simulink model "sumiao_zed"  (R2019a)
settings: Solver=FixedStepDiscrete  StartTime=0.0  StopTime=402*320  RelTol=1e-3
undefined symbols (not defined in the file): HDTV, Rec, SDTV
libraries: simulink x7, visionzynq_privlib x3, visionhdlutilities x3, dspvision x1, visionhdlconversions x1, visionsinks x1, visionzynqlib x1
settings Model: DataTypeOverride=Off  SimulationMode=accelerator  Creator=lbai  LastModifiedBy=lbai
settings DataIOCC: LimitDataPoints=on  SaveOutput=off  SignalLogging=off  DSMLogging=off  VisualizeSimOutput=off  SaveTime=off
settings OptimizationCC: BlockReduction=off  ConditionallyExecuteInputs=off  DefaultParameterBehavior=Inlined  LifeSpan=inf  SimCompilerOptimization=on
settings DebuggingCC: AlgebraicLoopMsg=error  SingleTaskRateTransMsg=error  ParameterPrecisionLossMsg=none  AllowSymbolicDim=off  PregeneratedLibrarySubsystemCodeDiagnostic=none  SFUnexpectedBacktrackingDiag=warning  SFNoUnconditionalDefaultTransitionDiag=warning  SFExecutionAtInitializationDiag=none  IntegerSaturationMsg=none  ArithmeticOperatorsInVariantConditions=warning
settings HardwareCC: ProdBitPerPointer=32  ProdBitPerSizeT=32  ProdBitPerPtrDiffT=32  ProdLargestAtomicFloat=None  ProdIntDivRoundTo=Undefined  ProdEndianess=Unspecified  ProdWordSize=32  ProdHWDeviceType=ASIC/FPGA->ASIC/FPGA  ProdEqTarget=off
settings SFSimCC: SimUseLocalCustomCode=off
settings RTWCC: RTWUseLocalCustomCode=off  BuildConfiguration=Faster Runs
settings CodeAppCC: StateflowObjectComments=on
settings GRTTargetCC: TargetLangStandard=C89/C90 (ANSI)  GeneratePreprocessorConditionals=Disable all
settings ConfigComp: CovMetricSettings=dw  CovHtmlReporting=on  CovSaveCumulativeToWorkspaceVar=on  CovSaveSingleToWorkspaceVar=on  CovExternalEMLEnable=off  CovSFcnEnable=off

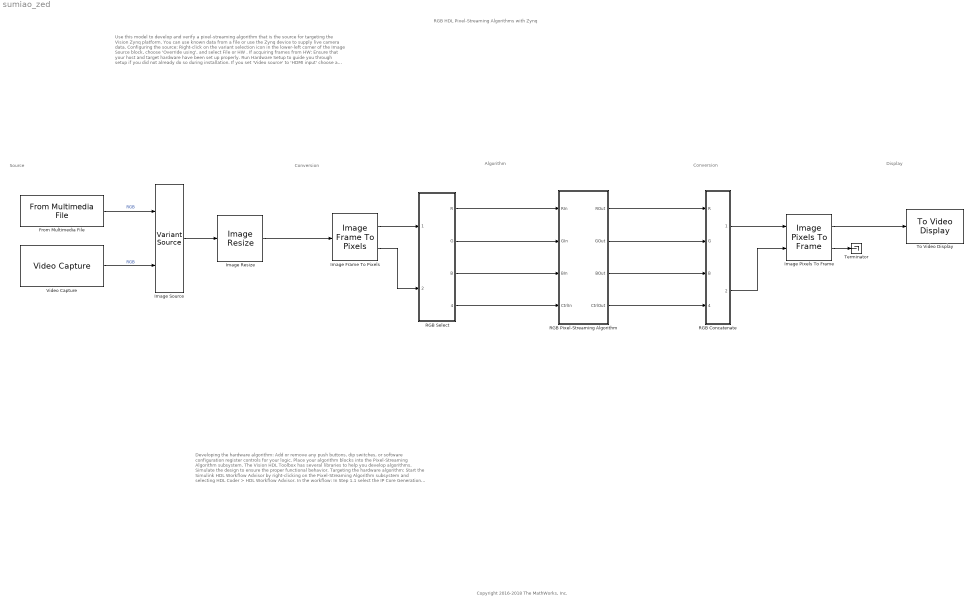
== system sumiao_zed ==
  note: Developing the hardware algorithm:
      | Add or remove any push buttons, dip switches, or software configuration register controls for your logic.
      | Place your algorithm blocks into the Pixel-Streaming Algorithm subsystem. The Vision HDL Toolbox has several libraries to help you develop algorithms.
      | Simulate the design to ensure the proper functional behavior.
      |
      | Targeting the hardware algorithm:
      |
      | Start the Simulink HDL Workflow Advisor by right-clicking on the Pixel-Streaming Algorithm subsystem and selecting HDL Coder > HDL Workflow Advisor.
      | In the workflow:
      | In Step 1.1 select the IP Core Generation workflow
      | In Step 1.1 select one of ZedBoard FMC-HDMI-CAM, ZC702 FMC-HDMI-CAM, ZC706 FMC-HDMI-CAM,
      | PicoZed FMC-HDMI-CAM.
      | In Step 1.2 select the reference platform that matches the desired pixel format.
      | In Step 1.3 map the reference design signals to the ports of the Pixel-Streaming Algorithm subsystem.
  note: Conversion
  note: Use this model to develop and verify a pixel-streaming algorithm that is the source for targeting the Vision Zynq platform. You can use known data from a file or use the Zynq device to supply live camera data.
      |
      | Configuring the source:
      | Right-click on the variant selection icon in the lower-left corner of the Image Source block, choose 'Override using', and select File or HW .
      | If acquiring frames from HW:
      | Ensure that your host and target hardware have been set up properly. Run Hardware Setup to guide you through setup if you did not already do so during installation.
      | If you set 'Video source' to 'HDMI input' choose a frame size that matches your camera settings.
      | If you set 'Video source' to 'Test pattern generator' choose any listed resolution. The hardware generates a color bar test pattern, and does not need an attached camera. It still requires the FMC board.
      | Since pixel-streaming algorithms will run many times slower than behavioral algorithms, consider adding a Resize block from Computer Vision System Toolbox to reduce the frame size that the algorithm operates on.
      |
      | Configuring conversions:
      | Ensure your Frame to Pixel and Pixel to Frame blocks match your source frame size.
  note: RGB HDL Pixel-Streaming Algorithms with Zynq
  note: Source
  note: Algorithm
  note: Display
  note: Conversion
  note: Copyright 2016-2018 The MathWorks, Inc.
  From Multimedia File : dspvision/From Multimedia File  inputFilename=vipbarcode.mp4  readRange=[1 Inf]  loop=on  numPlays=inf  outputStreams=Video only  videoDataType=uint8  audioDataType=int16  inheritSampleTime=off  userDefinedSampleTime=1/60  noAudioOutput=off  isIntensityVideo=off  fourcc=RGB  colorVideoFormat=One multidimensional signal  outputEOF=off  dataOrg=Column-major  audioFrameSize=1024  computeAudioFrameSize=off  outSamplingMode=Sample based
      settings: SourceProductName=DSP System Toolbox  SourceProductBaseCode=DS
  "Image Frame To Pixels " : visionzynq_privlib/Image Frame To Pixels   FrameSize=320x240p
      settings: SourceProductName=Computer Vision Toolbox Support Package for Xilinx Zynq-Based Hardware  SourceProductBaseCode=VP_VISION_ZYNQ
  Image Pixels To Frame : visionzynq_privlib/Image Pixels To Frame  FrameSize=320x240p
      settings: SourceProductName=Computer Vision Toolbox Support Package for Xilinx Zynq-Based Hardware  SourceProductBaseCode=VP_VISION_ZYNQ
  Image Resize : visionzynq_privlib/Image Resize  FrameSize=320x240p
      settings: SourceProductName=Computer Vision Toolbox Support Package for Xilinx Zynq-Based Hardware  SourceProductBaseCode=VP_VISION_ZYNQ
  Image Source : VariantSource  VariantControlMode=Label  LabelModeActiveChoice=File  ShowConditionOnBlock=on
  RGB Concatenate : Subsystem
  RGB Pixel-Streaming Algorithm : Subsystem  TreatAsAtomicUnit=on
  RGB Select : Subsystem
  Terminator : Terminator
  To Video Display : visionsinks/To Video Display  windowSizeMode=Normal  openAtMdlStart=on  fullScreen=off  videoWindowX=2182  videoWindowY=252  saveWindowSize=off  videoWindowWidth=926  videoWindowHeight=696  inputColorFormat=RGB  inputType=Obsolete  imagePorts=One multidimensional signal  OutputDevice=On-screen video monitor  dataOrg=Column-major  isWindowOpen=off
      settings: SourceProductName=Computer Vision Toolbox
  Video Capture : visionzynqlib/Video Capture  VideoSource=HDMI input  FrameSize=1080p HDTV (1920x1080p)  FrameRate=60fps  PixelFormatUI=RGB  CSCSpec=Rec. 709 (HDTV)  HWULBypass=off  CapturePoint=Input to FPGA user logic (A)  ROISource=No region of interest  ROIDimension=[100 100]  ROILocation=[1 1]  ImageSignal=One multidimensional signal  NoCameraHDMIMode=off  NoCameraHDMIColor=blue  CSCScanningStd=1125/60/2:1  TPGMode=Colorbars  TPGLevel=Line  TPGIncrement=bin2dec('0000')  EnablePixelFormat=on  MaskMode=Simulation
      settings: SourceProductName=Computer Vision Toolbox Support Package for Xilinx Zynq-Based Hardware  SourceProductBaseCode=VP_VISION_ZYNQ
  wires:
  "Image Frame To Pixels "/1 -> RGB Select/1(pixelData)
  "Image Frame To Pixels "/2 -> RGB Select/2(pixelCtrlIn)
  Image Pixels To Frame/2 -> Terminator/1
  Image Pixels To Frame/1 -> To Video Display/1
  RGB Concatenate/1(pixelData) -> Image Pixels To Frame/1
  RGB Concatenate/2(pixelCtrlOut) -> Image Pixels To Frame/2
  From Multimedia File/1 -> Image Source/1  "RGB"
  Video Capture/1 -> Image Source/2  "RGB"
  Image Source/1 -> Image Resize/1
  Image Resize/1 -> "Image Frame To Pixels "/1
  RGB Select/2(G) -> RGB Pixel-Streaming Algorithm/2(GIn)
  RGB Select/1(R) -> RGB Pixel-Streaming Algorithm/1(RIn)
  RGB Select/3(B) -> RGB Pixel-Streaming Algorithm/3(BIn)
  RGB Select/4(pixelCtrlOut) -> RGB Pixel-Streaming Algorithm/4(CtrlIn)
  RGB Pixel-Streaming Algorithm/1(ROut) -> RGB Concatenate/1(R)
  RGB Pixel-Streaming Algorithm/2(GOut) -> RGB Concatenate/2(G)
  RGB Pixel-Streaming Algorithm/3(BOut) -> RGB Concatenate/3(B)
  RGB Pixel-Streaming Algorithm/4(CtrlOut) -> RGB Concatenate/4(pixelCtrlIn)

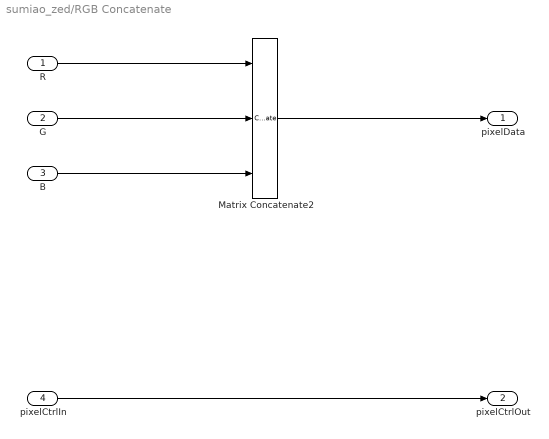
== system sumiao_zed/RGB Concatenate ==
  R : Inport
  G : Inport  Port=2
  B : Inport  Port=3
  pixelCtrlIn : Inport  Port=4
  Matrix Concatenate2 : Concatenate  NumInputs=3  Mode=Multidimensional array  ConcatenateDimension=2
  pixelData : Outport
  pixelCtrlOut : Outport  Port=2
  wires:
  R/1 -> Matrix Concatenate2/1
  G/1 -> Matrix Concatenate2/2
  Matrix Concatenate2/1 -> pixelData/1
  pixelCtrlIn/1 -> pixelCtrlOut/1
  B/1 -> Matrix Concatenate2/3

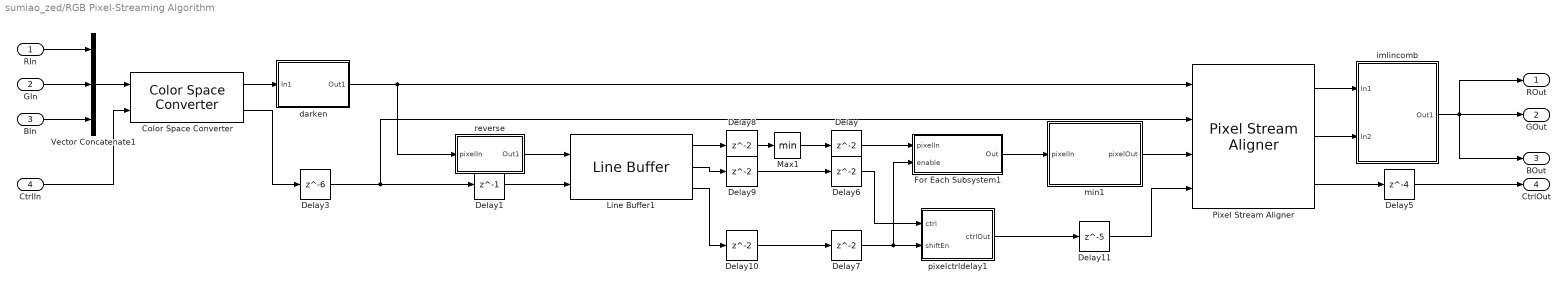
== system sumiao_zed/RGB Pixel-Streaming Algorithm ==
  RIn : Inport
  GIn : Inport  Port=2
  BIn : Inport  Port=3
  CtrlIn : Inport  Port=4
  Color Space Converter : visionhdlconversions/Color Space Converter  Conversion=RGB to intensity  ConversionStandard=Rec. 601 (SDTV)  ScanningStandard=1250/50/2:1  SimulateUsing=Code generation
      settings: SourceProductName=Vision HDL Toolbox  SourceProductBaseCode=VT
  Delay{,6..10} (6 alike) : Delay
  Delay1 : Delay  DelayLength=1
  Delay11 : Delay  DelayLength=5
  Delay3 : Delay  DelayLength=6
  Delay5 : Delay  DelayLength=4
  For Each Subsystem1 : Subsystem  TreatAsAtomicUnit=on
  Line Buffer1 : visionhdlutilities/Line Buffer  NeighborhoodSize=[3 3]  PaddingMethod=Symmetric  PaddingValue=0  LineBufferSize=2048  SimulateUsing=Code generation
      settings: SourceProductName=Vision HDL Toolbox  SourceProductBaseCode=VT
  Max1 : MinMax
  Pixel Stream Aligner : visionhdlutilities/Pixel Stream Aligner  LineBufferSize=2048  MaximumNumberOfLines=10  SimulateUsing=Code generation
      settings: SourceProductName=Vision HDL Toolbox  SourceProductBaseCode=VT
  Vector Concatenate1 : Concatenate  NumInputs=3  Mode=Multidimensional array  ConcatenateDimension=2
  darken : Subsystem
  imlincomb : Subsystem
  min1 : Subsystem
  pixelctrldelay1 : Subsystem
  reverse : Subsystem
  ROut : Outport
  GOut : Outport  Port=2
  BOut : Outport  Port=3
  CtrlOut : Outport  Port=4
  wires:
  Pixel Stream Aligner/1 -> imlincomb/1(In1)
  Pixel Stream Aligner/2 -> imlincomb/2(In2)
  Pixel Stream Aligner/3 -> Delay5/1
  Delay5/1 -> CtrlOut/1
  CtrlIn/1 -> Color Space Converter/2
  Color Space Converter/1 -> darken/1(In1)
  RIn/1 -> Vector Concatenate1/1
  GIn/1 -> Vector Concatenate1/2
  BIn/1 -> Vector Concatenate1/3
  imlincomb/1(Out1) -> ROut/1, BOut/1, GOut/1
  Vector Concatenate1/1 -> Color Space Converter/1
  Color Space Converter/2 -> Delay3/1
  For Each Subsystem1/1(Out) -> min1/1(pixelIn)
  Delay/1 -> For Each Subsystem1/1(pixelIn)
  min1/1(pixelOut) -> Pixel Stream Aligner/3
  Delay11/1 -> Pixel Stream Aligner/4
  Line Buffer1/1 -> Delay8/1
  Line Buffer1/2 -> Delay9/1
  Delay3/1 -> Pixel Stream Aligner/2, Delay1/1
  darken/1(Out1) -> Pixel Stream Aligner/1, reverse/1(pixelIn)
  Delay6/1 -> pixelctrldelay1/1(ctrl)
  Delay7/1 -> For Each Subsystem1/2(enable), pixelctrldelay1/2(shiftEn)
  reverse/1(Out1) -> Line Buffer1/1
  Delay8/1 -> Max1/1
  Delay9/1 -> Delay6/1
  Delay1/1 -> Line Buffer1/2
  Delay10/1 -> Delay7/1
  Line Buffer1/3 -> Delay10/1
  Max1/1 -> Delay/1
  pixelctrldelay1/1(ctrlOut) -> Delay11/1

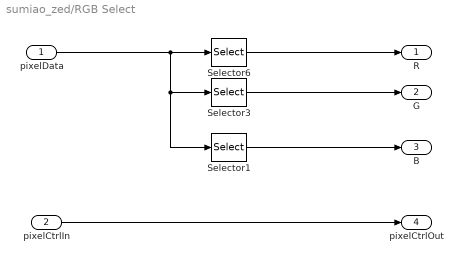
== system sumiao_zed/RGB Select ==
  pixelData : Inport
  pixelCtrlIn : Inport  Port=2
  Selector1 : Selector  NumberOfDimensions=2  InputPortWidth=3  IndexOptions=Select all,Index vector (dialog)  Indices=[1 3],3  OutputSizes=1,1
  Selector3 : Selector  NumberOfDimensions=2  InputPortWidth=3  IndexOptions=Select all,Index vector (dialog)  Indices=[1 3],2  OutputSizes=1,1
  Selector6 : Selector  NumberOfDimensions=2  InputPortWidth=3  IndexOptions=Select all,Index vector (dialog)  Indices=[1 3],1  OutputSizes=1,1
  R : Outport
  G : Outport  Port=2
  B : Outport  Port=3
  pixelCtrlOut : Outport  Port=4
  wires:
  pixelData/1 -> Selector1/1, Selector3/1, Selector6/1
  pixelCtrlIn/1 -> pixelCtrlOut/1
  Selector3/1 -> G/1
  Selector6/1 -> R/1
  Selector1/1 -> B/1

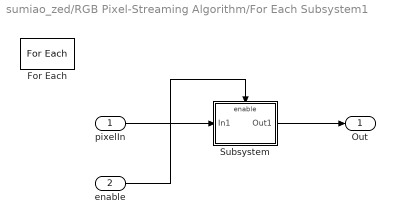
== system sumiao_zed/RGB Pixel-Streaming Algorithm/For Each Subsystem1 ==
  pixelIn : Inport  Partition=on  PartitionDimension=1  PartitionWidth=1  PartitionOffset=0
  enable : Inport  Port=2
  For Each : ForEach  DisableCoverage=on
  Subsystem : Subsystem
  Out : Outport  ConcatenationDimension=1  VectorParamsAs1DForOutWhenUnconnected=on
  wires:
  enable/1 -> Subsystem/Enable
  Subsystem/1(Out1) -> Out/1
  pixelIn/1 -> Subsystem/1(In1)

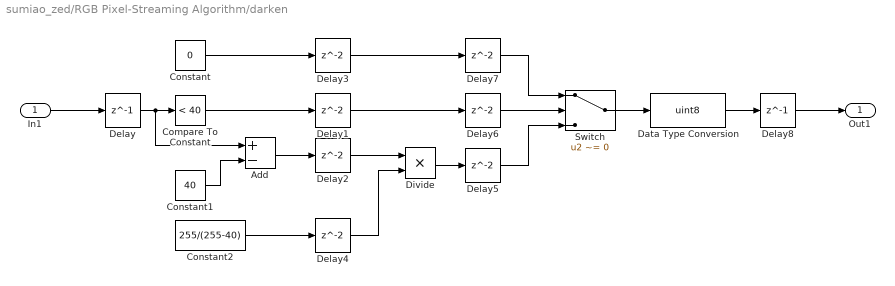
== system sumiao_zed/RGB Pixel-Streaming Algorithm/darken ==
  In1 : Inport
  Add : Sum  Inputs=+-
  Compare To Constant : simulink/Logic and Bit Operations/Compare To Constant  relop=<  const=40  OutDataTypeStr=boolean
  Constant : Constant  Value=0  OutDataTypeStr=uint8  SampleTime=-1
  Constant1 : Constant  Value=40  OutDataTypeStr=uint8  SampleTime=-1
  Constant2 : Constant  Value=255/(255-40)  OutDataTypeStr=fixdt(0,16,15)  SampleTime=-1
  Data Type Conversion : DataTypeConversion  OutDataTypeStr=uint8  RndMeth=Round
  Delay : Delay  DelayLength=1
  Delay{1..7} (7 alike) : Delay
  Delay8 : Delay  DelayLength=1
  Divide : Product  Inputs=**
  Switch : Switch  Criteria=u2 ~= 0
  Out1 : Outport  VectorParamsAs1DForOutWhenUnconnected=on
  wires:
  Delay4/1 -> Divide/2
  Delay2/1 -> Divide/1
  Delay6/1 -> Switch/2
  Constant1/1 -> Add/2
  Delay/1 -> Compare To Constant/1, Add/1
  Switch/1 -> Data Type Conversion/1
  Delay1/1 -> Delay6/1
  Constant/1 -> Delay3/1
  Compare To Constant/1 -> Delay1/1
  Divide/1 -> Delay5/1
  Delay7/1 -> Switch/1
  Constant2/1 -> Delay4/1
  Delay5/1 -> Switch/3
  Delay8/1 -> Out1/1
  Delay3/1 -> Delay7/1
  Add/1 -> Delay2/1
  In1/1 -> Delay/1
  Data Type Conversion/1 -> Delay8/1

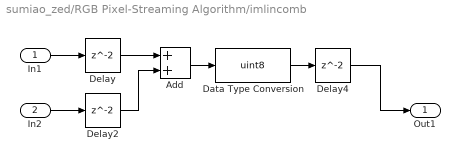
== system sumiao_zed/RGB Pixel-Streaming Algorithm/imlincomb ==
  In1 : Inport
  In2 : Inport  Port=2
  Add : Sum
  Data Type Conversion : DataTypeConversion  OutDataTypeStr=uint8
  Delay : Delay
  Delay2 : Delay
  Delay4 : Delay
  Out1 : Outport  VectorParamsAs1DForOutWhenUnconnected=on
  wires:
  Delay4/1 -> Out1/1
  Delay/1 -> Add/1
  Add/1 -> Data Type Conversion/1
  Delay2/1 -> Add/2
  Data Type Conversion/1 -> Delay4/1
  In1/1 -> Delay/1
  In2/1 -> Delay2/1

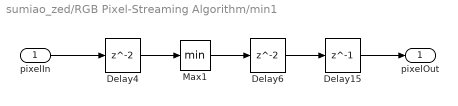
== system sumiao_zed/RGB Pixel-Streaming Algorithm/min1 ==
  pixelIn : Inport
  Delay15 : Delay  DelayLength=1
  Delay4 : Delay
  Delay6 : Delay
  Max1 : MinMax
  pixelOut : Outport  VectorParamsAs1DForOutWhenUnconnected=on
  wires:
  Delay6/1 -> Delay15/1
  Delay15/1 -> pixelOut/1
  Max1/1 -> Delay6/1
  pixelIn/1 -> Delay4/1
  Delay4/1 -> Max1/1

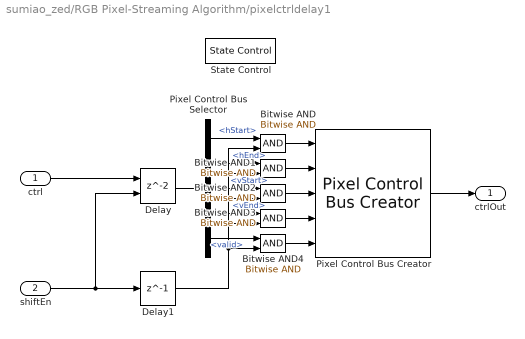
== system sumiao_zed/RGB Pixel-Streaming Algorithm/pixelctrldelay1 ==
  ctrl : Inport
  shiftEn : Inport  Port=2
  Bitwise AND{,1..4} (5 alike) : simulink/Logic and Bit Operations/Bitwise Operator  logicop=AND  UseBitMask=off  NumInputPorts=2  BitMask=bin2dec('11011001')  BitMaskRealWorld=Stored Integer
  Delay : Delay  ShowEnablePort=on
      settings: InputPortMap=u0,e6
  Delay1 : Delay  DelayLength=1
  Pixel Control Bus Creator : visionhdlutilities/Pixel Control Bus Creator
      settings: SourceProductName=Vision HDL Toolbox  SourceProductBaseCode=VT
  Pixel Control Bus Selector : BusSelector  OutputSignals=hStart,hEnd,vStart,vEnd,valid
  State Control : StateControl  StateControl=Synchronous
  ctrlOut : Outport
  wires:
  Delay1/1 -> Bitwise AND4/2, Bitwise AND/2, Bitwise AND1/2, Bitwise AND2/2, Bitwise AND3/2
  shiftEn/1 -> Delay/2, Delay1/1
  ctrl/1 -> Delay/1
  Pixel Control Bus Creator/1 -> ctrlOut/1
  Bitwise AND1/1 -> Pixel Control Bus Creator/2
  Pixel Control Bus Selector/4 -> Bitwise AND3/1  "<vEnd>"
  Bitwise AND2/1 -> Pixel Control Bus Creator/3
  Pixel Control Bus Selector/2 -> Bitwise AND1/1  "<hEnd>"
  Pixel Control Bus Selector/1 -> Bitwise AND/1  "<hStart>"
  Delay/1 -> Pixel Control Bus Selector/1
  Pixel Control Bus Selector/5 -> Bitwise AND4/1  "<valid>"
  Bitwise AND3/1 -> Pixel Control Bus Creator/4
  Pixel Control Bus Selector/3 -> Bitwise AND2/1  "<vStart>"
  Bitwise AND/1 -> Pixel Control Bus Creator/1
  Bitwise AND4/1 -> Pixel Control Bus Creator/5

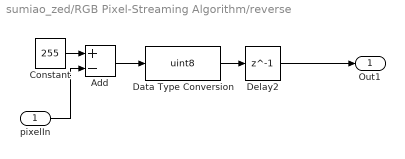
== system sumiao_zed/RGB Pixel-Streaming Algorithm/reverse ==
  pixelIn : Inport
  Add : Sum  Inputs=+-
  Constant : Constant  Value=255  OutDataTypeStr=uint8
  Data Type Conversion : DataTypeConversion  OutDataTypeStr=uint8
  Delay2 : Delay  DelayLength=1
  Out1 : Outport  VectorParamsAs1DForOutWhenUnconnected=on
  wires:
  pixelIn/1 -> Add/2
  Constant/1 -> Add/1
  Data Type Conversion/1 -> Delay2/1
  Add/1 -> Data Type Conversion/1
  Delay2/1 -> Out1/1

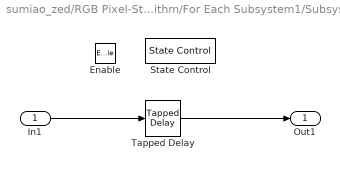
== system sumiao_zed/RGB Pixel-Streaming Algorithm/For Each Subsystem1/Subsystem ==
  In1 : Inport
  Enable : EnablePort
  State Control : StateControl  StateControl=Synchronous
  Tapped Delay : simulink/Discrete/Tapped Delay  vinit=0.0  samptime=-1  NumDelays=3  DelayOrder=Oldest  includeCurrent=off
  Out1 : Outport  VectorParamsAs1DForOutWhenUnconnected=on
  wires:
  Tapped Delay/1 -> Out1/1
  In1/1 -> Tapped Delay/1
